simulink model "dbl_pend_upup_stab_RL_simulink"  (R2023a)
settings: Solver=VariableStepAuto  StartTime=0.0  StopTime=10  RelTol=1e-3
values from neighbouring files (symbols this model uses):
  b1 = 7.7210    (= 7.721)    [benchmark_dbl_pend.m]    (also in dbl_pend_upup_stab_RL.m = 4.8)
  b2 = 2.337424773114795e-05    (= 2.33742477311e-05)    [benchmark_dbl_pend.m]    (also in dbl_pend_upup_stab_RL.m = 0.0002)
  bounds_th1 = [-pi, 3*pi]    [dbl_pend_upup_stab_RL.m]
  c1 = -0.0320    (= -0.032)    [benchmark_dbl_pend.m]    (also in dbl_pend_upup_stab_RL.m = -0.04)
  c2 = 0.053232610186913    (= 0.0532326101869)    [benchmark_dbl_pend.m]    (also in dbl_pend_upup_stab_RL.m = 0.06)
  I1 = 0.0888    [benchmark_dbl_pend.m]    (also in dbl_pend_upup_stab_RL.m = 0.074)
  I2 = 9.5326e-05    [benchmark_dbl_pend.m]    (also in dbl_pend_upup_stab_RL.m = 0.00012)
  init_cond = [0.1, -0.1, 0, 0]    [benchmark_dbl_pend.m]    (also in dbl_pend_upup_stab_RL.m = [pi, 0, 0, 0])
  km = 53.049364666321930    (= 53.0493646663)    [benchmark_dbl_pend.m]    (also in dbl_pend_upup_stab_RL.m = 50)
  l1 = 0.1    [benchmark_dbl_pend.m]    (also in dbl_pend_upup_stab_RL.m)
  l2 = 0.1    [benchmark_dbl_pend.m]    (also in dbl_pend_upup_stab_RL.m)
  m1 = 0.125    [benchmark_dbl_pend.m]    (also in dbl_pend_upup_stab_RL.m)
  m2 = 0.0493    [benchmark_dbl_pend.m]    (also in dbl_pend_upup_stab_RL.m = 0.05)
  tau_e = 0.014999999999983    (= 0.015)    [benchmark_dbl_pend.m]    (also in dbl_pend_upup_stab_RL.m = 0.03)
  w = [1, 1, 0.05, 0.1]    [dbl_pend_upup_stab_RL.m]
libraries: simulink x5, rllib x1
settings Model: Creator=MICHAEL-LT  LastModifiedBy=Michael
settings DebuggingCC: UnconnectedInputMsg=warning  UnconnectedOutputMsg=warning  UnconnectedLineMsg=warning
settings ModelReferenceCC: EnableRefExpFcnMdlSchedulingChecks=on
settings RTWCC: DLArmComputeVersion=19.05

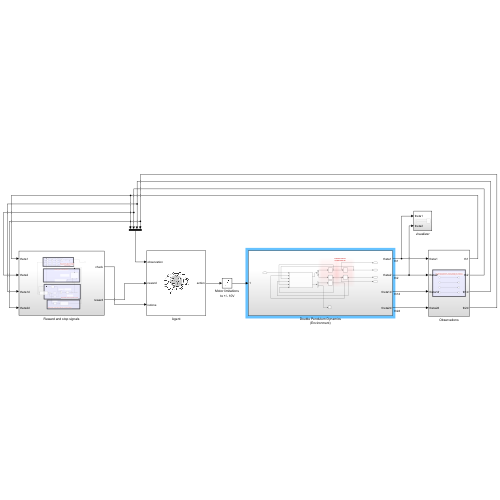
[thumbnail: Simulink's stored preview of the top-level diagram]
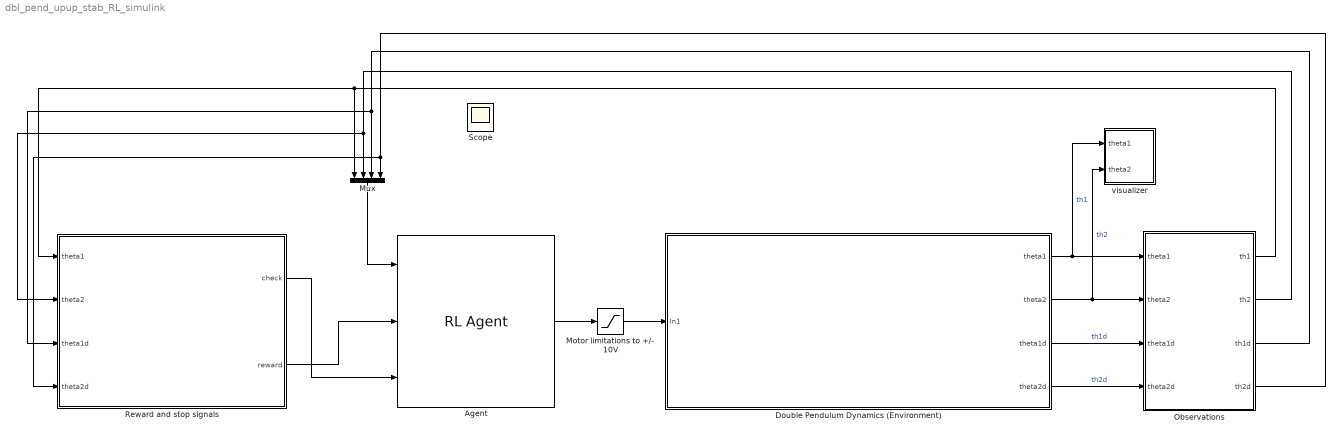
== system dbl_pend_upup_stab_RL_simulink ==
  Agent : rllib/RL Agent  Agent=agent  ExternalActionAsInput=off  ProvideLastAction=off  ProvideCumRwd=off  TreatAsDirectFeedthrough=on  UseStrictObservationDataTypes=off
  Double Pendulum Dynamics (Environment) : Subsystem
  Motor limitations to +/- 10V : Saturate  UpperLimit=10  LowerLimit=-10
  Mux : Mux
  Observations : Subsystem
  Reward and stop signals : Subsystem
  visualizer : Subsystem
  Scope : Scope
  wires:
  Double Pendulum Dynamics (Environment)/2(theta2) -> visualizer/2(theta2), Observations/2(theta2)  "th2"
  Double Pendulum Dynamics (Environment)/3(theta1d) -> Observations/3(theta1d)  "th1d"
  Double Pendulum Dynamics (Environment)/1(theta1) -> visualizer/1(theta1), Observations/1(theta1)  "th1"
  Double Pendulum Dynamics (Environment)/4(theta2d) -> Observations/4(theta2d)  "th2d"
  Observations/2(th2) -> Mux/2, Reward and stop signals/2(theta2)
  Observations/3(th1d) -> Mux/3, Reward and stop signals/3(theta1d)
  Observations/1(th1) -> Mux/1, Reward and stop signals/1(theta1)
  Observations/4(th2d) -> Mux/4, Reward and stop signals/4(theta2d)
  Reward and stop signals/2(reward) -> Agent/2
  Mux/1 -> Agent/1
  Agent/1 -> Motor limitations to +/- 10V/1
  Motor limitations to +/- 10V/1 -> Double Pendulum Dynamics (Environment)/1(In1)
  Reward and stop signals/1(check) -> Agent/3

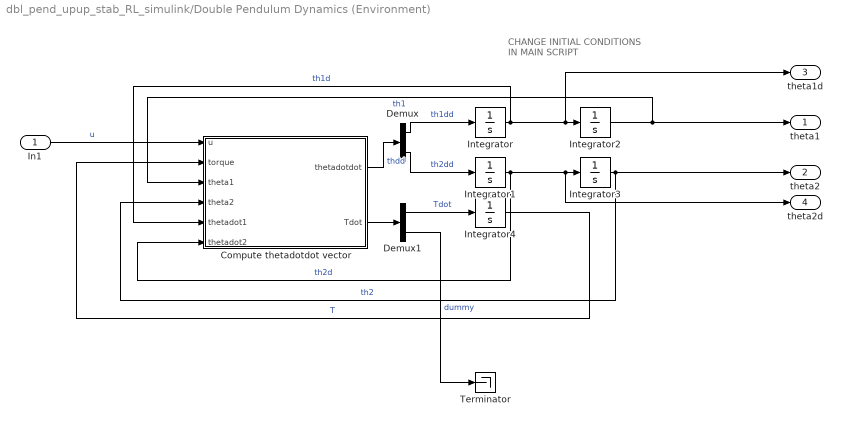
== system dbl_pend_upup_stab_RL_simulink/Double Pendulum Dynamics (Environment) ==
  note: CHANGE INITIAL CONDITIONS IN MAIN SCRIPT
  In1 : Inport
  Compute thetadotdot vector : MATLAB Function  TreatAsAtomicUnit=on
  Demux : Demux  Outputs=2
  Demux1 : Demux  Outputs=2
  Integrator : Integrator  InitialCondition=init_cond(3)
  Integrator1 : Integrator  InitialCondition=init_cond(4)
  Integrator2 : Integrator  InitialCondition=init_cond(1)
  Integrator3 : Integrator  InitialCondition=init_cond(2)
  Integrator4 : Integrator
  Terminator : Terminator
  theta1 : Outport
  theta2 : Outport  Port=2
  theta1d : Outport  Port=3
  theta2d : Outport  Port=4
  wires:
  Integrator1/1 -> Compute thetadotdot vector/6(thetadot2), theta2d/1, Integrator3/1  "th2d"
  Integrator4/1 -> Compute thetadotdot vector/2(torque)  "T"
  Demux1/2 -> Terminator/1  "dummy"
  Compute thetadotdot vector/2(Tdot) -> Demux1/1
  In1/1 -> Compute thetadotdot vector/1(u)  "u"
  Compute thetadotdot vector/1(thetadotdot) -> Demux/1  "thdd"
  Integrator/1 -> Compute thetadotdot vector/5(thetadot1), theta1d/1, Integrator2/1  "th1d"
  Integrator3/1 -> theta2/1, Compute thetadotdot vector/4(theta2)  "th2"
  Demux1/1 -> Integrator4/1  "Tdot"
  Integrator2/1 -> Compute thetadotdot vector/3(theta1), theta1/1  "th1"
  Demux/2 -> Integrator1/1  "th2dd"
  Demux/1 -> Integrator/1  "th1dd"

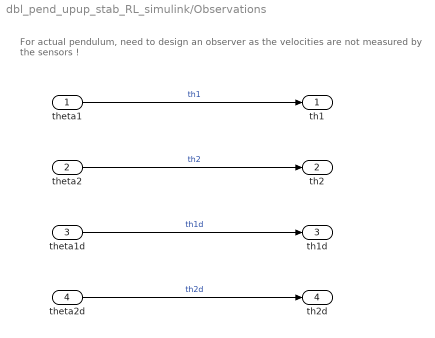
== system dbl_pend_upup_stab_RL_simulink/Observations ==
  note: For actual pendulum, need to design an observer
      | as the velocities are not measured by the sensors !
  theta1 : Inport
  theta2 : Inport  Port=2
  theta1d : Inport  Port=3
  theta2d : Inport  Port=4
  th1 : Outport
  th2 : Outport  Port=2
  th1d : Outport  Port=3
  th2d : Outport  Port=4
  wires:
  theta1/1 -> th1/1  "th1"
  theta2/1 -> th2/1  "th2"
  theta1d/1 -> th1d/1  "th1d"
  theta2d/1 -> th2d/1  "th2d"

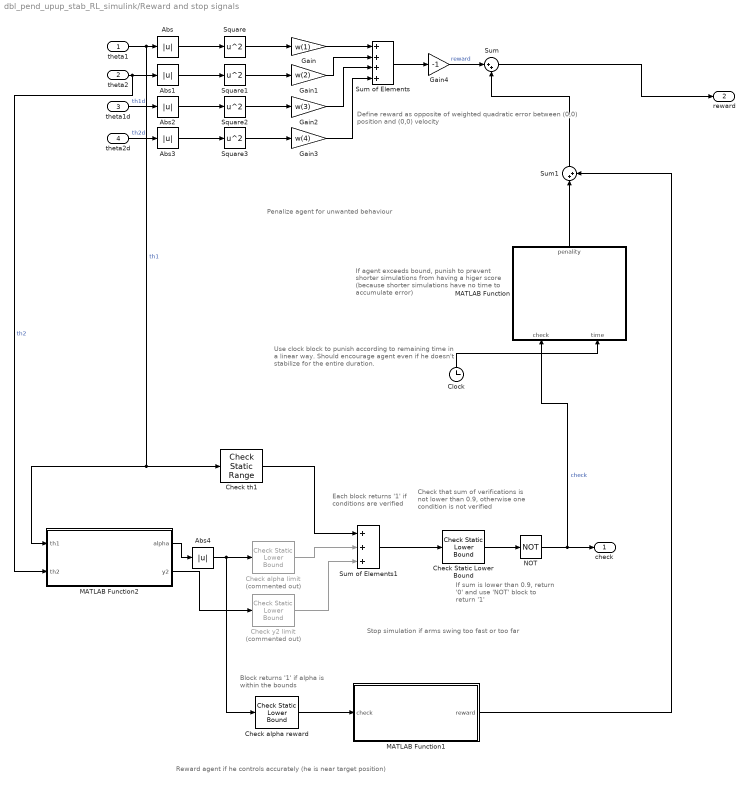
== system dbl_pend_upup_stab_RL_simulink/Reward and stop signals ==
  note: Block returns '1' if alpha
      | is within the bounds
  note: Each block returns '1'
      | if conditions are verified
  note: Define reward as opposite of weighted
      | quadratic error between (0,0) position
      | and (0,0) velocity
  note: Stop simulation if arms swing too fast or too far
  note: Check that sum of verifications
      | is not lower than 0.9, otherwise
      | one condition is not verified
  note: If sum is lower than 0.9,
      | return '0' and use 'NOT' block
      | to return '1'
  note: If agent exceeds bound, punish
      | to prevent shorter simulations from having
      | a higer score (because shorter simulations
      | have no time to accumulate error)
  note: Penalize agent for unwanted behaviour
  note: Use clock block to punish according to remaining time
      | in a linear way. Should encourage agent even if he
      | doesn't stabilize for the entire duration.
  note: Reward agent if he controls accurately (he is near target position)
  theta1 : Inport
  theta2 : Inport  Port=2
  theta1d : Inport  Port=3
  theta2d : Inport  Port=4
  Abs{,1..4} (5 alike) : Abs  SaturateOnIntegerOverflow=off
  Check Static Lower Bound : simulink/Model Verification/Check Static  Lower Bound  Description=0.9 <= u  min=0.9  min_included=on  enabled=on  stopWhenAssertionFail=off  export=on  icon=graphic
  Check alpha limit : simulink/Model Verification/Check Static  Lower Bound  Description=bounds_alpha_limit <= u  Commented=on  min=bounds_alpha_limit  min_included=on  enabled=on  callback="fprintf(\"Bounds exceeded on alpha ! Simulation stopped...\")"  stopWhenAssertionFail=off  export=on  icon=graphic
  Check alpha reward : simulink/Model Verification/Check Static  Lower Bound  Description=bounds_alpha_reward <= u  min=bounds_alpha_reward  min_included=on  enabled=on  stopWhenAssertionFail=off  export=on  icon=graphic
  Check th1 : simulink/Model Verification/Check  Static Range  Description=bounds_th1(1) <= u <= bounds_th1(2)  max=bounds_th1(2)  max_included=on  min=bounds_th1(1)  min_included=on  enabled=on  callback="fprintf(\"Bounds exceeded on theta1 ! Simulation stopped...\")"  stopWhenAssertionFail=off  export=on  icon=graphic
  Check y2 limit : simulink/Model Verification/Check Static  Lower Bound  Description=0.75*(l1 + l2) <= u  Commented=on  min=0.75*(l1 + l2)  min_included=on  enabled=on  callback="fprintf(\"Bounds exceeded on alpha ! Simulation stopped...\")"  stopWhenAssertionFail=off  export=on  icon=graphic
  Clock : Clock
  Gain : Gain  Gain=w(1)
  Gain1 : Gain  Gain=w(2)
  Gain2 : Gain  Gain=w(3)
  Gain3 : Gain  Gain=w(4)
  Gain4 : Gain  Gain=-1
  MATLAB Function : MATLAB Function  TreatAsAtomicUnit=on
  MATLAB Function1 : MATLAB Function  TreatAsAtomicUnit=on
  MATLAB Function2 : MATLAB Function  TreatAsAtomicUnit=on
  NOT : Logic  Operator=NOT  IconShape=distinctive  AllPortsSameDT=off  OutDataTypeStr=boolean
  Square{,1..3} (4 alike) : Math  Operator=square
  Sum : Sum  Inputs=|++
  Sum of Elements : Sum  Inputs=++++
  Sum of Elements1 : Sum  Inputs=+++
  Sum1 : Sum  Inputs=|++
  check : Outport
  reward : Outport  Port=2
  wires:
  Square/1 -> Gain/1
  Square1/1 -> Gain1/1
  Square2/1 -> Gain2/1
  Square3/1 -> Gain3/1
  theta2d/1 -> Abs3/1  "th2d"
  theta1d/1 -> Abs2/1  "th1d"
  theta2/1 -> MATLAB Function2/2(th2), Abs1/1  "th2"
  theta1/1 -> MATLAB Function2/1(th1), Check th1/1, Abs/1  "th1"
  Abs/1 -> Square/1
  Abs1/1 -> Square1/1
  Abs2/1 -> Square2/1
  Abs3/1 -> Square3/1
  Gain/1 -> Sum of Elements/1
  Gain1/1 -> Sum of Elements/2
  Gain2/1 -> Sum of Elements/3
  Gain3/1 -> Sum of Elements/4
  Sum of Elements/1 -> Gain4/1
  Check th1/1 -> Sum of Elements1/1
  Sum of Elements1/1 -> Check Static Lower Bound/1
  Check Static Lower Bound/1 -> NOT/1
  NOT/1 -> check/1, MATLAB Function/1(check)  "check"
  Check alpha limit/1 -> Sum of Elements1/2
  Clock/1 -> MATLAB Function/2(time)
  Gain4/1 -> Sum/1  "reward"
  Sum/1 -> reward/1
  Check alpha reward/1 -> MATLAB Function1/1(check)
  MATLAB Function/1(penality) -> Sum1/1
  Sum1/1 -> Sum/2
  MATLAB Function1/1(reward) -> Sum1/2
  MATLAB Function2/1(alpha) -> Abs4/1
  Abs4/1 -> Check alpha reward/1, Check alpha limit/1
  MATLAB Function2/2(y2) -> Check y2 limit/1
  Check y2 limit/1 -> Sum of Elements1/3

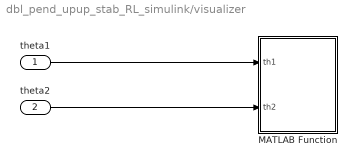
== system dbl_pend_upup_stab_RL_simulink/visualizer ==
  theta1 : Inport
  theta2 : Inport  Port=2
  MATLAB Function : MATLAB Function  TreatAsAtomicUnit=on
  wires:
  theta1/1 -> MATLAB Function/1(th1)
  theta2/1 -> MATLAB Function/2(th2)

== matlab function dbl_pend_upup_stab_RL_simulink/visualizer/MATLAB Function ==
  settings: updateMethod=DISCRETE
  data: th1 input; th2 input; l1 parameter; l2 parameter
function plotSituation(th1, th2, l1, l2)
coder.extrinsic('plotDoublePend');
plotDoublePend(th1, th2, l1, l2);

== matlab function dbl_pend_upup_stab_RL_simulink/Double Pendulum Dynamics (Environment)/Compute thetadotdot vector ==
  data: u input; torque input; thetadotdot output; theta1 input; theta2 input; thetadot1 input; thetadot2 input; l1 parameter; l2 parameter; m1 parameter; m2 parameter; c1 parameter; c2 parameter; I1 parameter; I2 parameter; b1 parameter; b2 parameter; km parameter; Tdot output; tau_e parameter
function [thetadotdot, Tdot]  = get_thetadotdot(u, torque, theta1, theta2, thetadot1, thetadot2, l1, l2, m1, m2, c1, c2, I1, I2, b1, b2, km, tau_e)
%% Parameters (SI Units)
g = 9.81;
%% Variables of the model
th1 = theta1;
th2 = theta2;
th1d = thetadot1;
th2d = thetadot2;
thd_vec = [th1d ; th2d];
thetadotdot = [0 ; 0];
T_vec = [torque, 0];

%% Matrices of physical model
P1 = m1 * c1 * c1 + m2 * l1 * l1 + I1;
P2 = m2 * c2 * c2 + I2;
P3 = m2 * l1 * c2;
g1 = (m1 * c1 + m2 * l1) * g;
g2 = m2 * c2 * g;

M = [[P1 + P2 + 2*P3*cos(th2), P2 + P3 * cos(th2)]; [P2 + P3 * cos(th2) P2]];
C = [[b1 - P3 * th2d * sin(th2), -P3 * (th1d + th2d)*sin(th2)]; [P3 * th1d * sin(th2), b2]];
G = [- g1 * sin(th1) - g2 * sin(th1 + th2); - g2 * sin(th1 + th2)];

%% Compute output angular acceleration
M_inv = inv(M);
Tdot = (km*u - T_vec)/tau_e;
thetadotdot = M_inv*T_vec - M_inv*C*thd_vec - M_inv*G;

== matlab function dbl_pend_upup_stab_RL_simulink/Reward and stop signals/MATLAB Function ==
  data: check input; penality output; time input; T_final parameter
function penality = PunishAgentIfExceedBounds(check, time, T_final)
penality = 0;
timePercentageNotAccomplished = 1 - time/T_final;
maxPenality = -10000;
if check
    penality = -100000 + timePercentageNotAccomplished*maxPenality;
end

== matlab function dbl_pend_upup_stab_RL_simulink/Reward and stop signals/MATLAB Function1 ==
  data: check input; reward output
function reward = RewardAgentIfWithinBounds(check)
reward = 0;
if check
    reward = 100;
end

== matlab function dbl_pend_upup_stab_RL_simulink/Reward and stop signals/MATLAB Function2 ==
  data: th1 input; alpha output; l1 parameter; l2 parameter; th2 input; y2 output
function [alpha, y2] = ComputeAnglesAndPositions(th1, l1, l2, th2)
% Function that computes angle 'alpha' between second mass and horizontal axis.
% Input: 'th1' -> angle theta1 of first mass with horizontal axis in radians. Positive to the right.
% Input: 'th2' -> angle theta2 of second mass with first arm in radians. Positive to the left.
% Parameter: 'l1' -> length of first arm in meters. Must be positive. 
% Parameter: 'l2' -> length of second arm in meters. Must be positive.
% Output: 'alpha' -> angle between second mass and horizontal axis in radians. Is within -pi/2 (upper left quadrant) and pi/2 (upper right quadrant).

x1 = l1 * sin(th1);
y1 = l1 * cos(th1);
x2 = x1 + l2*sin(th1 + th2);
y2 = y1 + l2*cos(th1 + th2);

alpha = atan(y2/x2);
